simulink model "control_pos_6dof_sinMI"  (R2023b)
settings: Solver=ode45  StartTime=0.0  StopTime=tsim  FixedStep=tstep  MaxStep=tstep  RelTol=tstep/10
undefined symbols (not defined in the file): a0, a1, robot_params, t_qeq_init, t_tr_init, tau_L, tr_ref
(part 7 of 7)

== matlab function control_pos_6dof_sinMI/q to xyz (robot)/q to xyz ==
  data: robot_params input; p output size=[3,6]; q input size=[6,1]; dq input size=[6,1]; ddq input size=[6,1]; dp output size=[3,1]; ddp output size=[3,1]
function [p,dp,ddp] = fcn(robot_params,q,dq,ddq)

l1 = robot_params.l(1);
l2 = robot_params.l(2);
l3 = robot_params.l(3);
l4 = robot_params.l(4);
l5 = robot_params.l(5);
l6 = robot_params.l(6);

lc1 = robot_params.lc(1);
lc2 = robot_params.lc(2);
lc3 = robot_params.lc(3);
lc4 = robot_params.lc(4);
lc5 = robot_params.lc(5);
lc6 = robot_params.lc(6);

d1 = robot_params.d(1);
d2 = robot_params.d(2);
d3 = robot_params.d(3);
d4 = robot_params.d(4);
d5 = robot_params.d(5);
d6 = robot_params.d(6);

dc1 = robot_params.dc(1);
dc2 = robot_params.dc(2);
dc3 = robot_params.dc(3);
dc4 = robot_params.dc(4);
dc5 = robot_params.dc(5);
dc6 = robot_params.dc(6);

q1 = q(1);
q2 = q(2);
q3 = q(3);
q4 = q(4);
q5 = q(5);
q6 = q(6);


% Cinematica directa %%%%%%%%%%%%%%%%%%%%%%%%%%%%%%%%%%%%%%%%%%%%%%%%%%%%%%

DH = [0   pi/2  d1 q1;
      l2  0     0  q2;
      l3  0     0  q3;
      0   pi/2  d4 q4;
      0   -pi/2 d5 q5;
      0   0     d6 q6];

A01 = transformacion_homogenea(DH(1,:));
A12 = transformacion_homogenea(DH(2,:));
A23 = transformacion_homogenea(DH(3,:));
A34 = transformacion_homogenea(DH(4,:));
A45 = transformacion_homogenea(DH(5,:));
A56 = transformacion_homogenea(DH(6,:));

T0 = zeros(4,4,6);

T0(:,:,1) = A01;
T0(:,:,2) = A01*A12;
T0(:,:,3) = A01*A12*A23;
T0(:,:,4) = A01*A12*A23*A34;
T0(:,:,5) = A01*A12*A23*A34*A45;
T0(:,:,6) = A01*A12*A23*A34*A45*A56;

p = reshape(T0(1:3,4,:),[3,6]);


% Cinematica diferencial %%%%%%%%%%%%%%%%%%%%%%%%%%%%%%%%%%%%%%%%%%%%%%%%%%
JP = zeros(3,6);

JP(1,1) = -cos(q1)*(d1 + l3*sin(q2 + q3) + l2*sin(q2) - d5*cos(q2 + q3 + q4) - dc6*sin(q2 + q3 + q4)*sin(q5));
JP(1,2) = -cos(q1)*(d1 - dc1 + l3*sin(q2 + q3) + l2*sin(q2) - d5*cos(q2 + q3 + q4) - dc6*sin(q2 + q3 + q4)*sin(q5));
JP(1,3) = cos(q1)*(lc2*sin(q2) - l2*sin(q2) - l3*sin(q2 + q3) + d5*cos(q2 + q3 + q4) + dc6*sin(q2 + q3 + q4)*sin(q5));
JP(1,4) = - cos(q2 + q3 + q4)*(dc6*(cos(q1)*cos(q5) + cos(q2 + q3 + q4)*sin(q1)*sin(q5)) + d4*cos(q1) - sin(q1)*(l3*cos(q2 + q3) + l2*cos(q2)) + sin(q1)*(lc3*cos(q2 + q3) + l2*cos(q2)) - d5*sin(q2 + q3 + q4)*sin(q1)) - sin(q2 + q3 + q4)*sin(q1)*(lc3*sin(q2 + q3) - l3*sin(q2 + q3) + d5*cos(q2 + q3 + q4) + dc6*sin(q2 + q3 + q4)*sin(q5));
JP(1,5) = d5*sin(q1)*sin(q5) + d5*cos(q2 + q3 + q4)*cos(q1)*cos(q5) - d4*sin(q2 + q3 + q4)*cos(q1)*sin(q5) + dc4*sin(q2 + q3 + q4)*cos(q1)*sin(q5);
JP(1,6) = (d5 - dc5)*(sin(q1)*sin(q5) + cos(q2 + q3 + q4)*cos(q1)*cos(q5));

JP(2,1) = -sin(q1)*(d1 + l3*sin(q2 + q3) + l2*sin(q2) - d5*cos(q2 + q3 + q4) - dc6*sin(q2 + q3 + q4)*sin(q5));
JP(2,2) = -sin(q1)*(d1 - dc1 + l3*sin(q2 + q3) + l2*sin(q2) - d5*cos(q2 + q3 + q4) - dc6*sin(q2 + q3 + q4)*sin(q5));
JP(2,3) = sin(q1)*(lc2*sin(q2) - l2*sin(q2) - l3*sin(q2 + q3) + d5*cos(q2 + q3 + q4) + dc6*sin(q2 + q3 + q4)*sin(q5));
JP(2,4) = sin(q2 + q3 + q4)*cos(q1)*(lc3*sin(q2 + q3) - l3*sin(q2 + q3) + d5*cos(q2 + q3 + q4) + dc6*sin(q2 + q3 + q4)*sin(q5)) - cos(q2 + q3 + q4)*(dc6*(cos(q5)*sin(q1) - cos(q2 + q3 + q4)*cos(q1)*sin(q5)) + cos(q1)*(l3*cos(q2 + q3) + l2*cos(q2)) - cos(q1)*(lc3*cos(q2 + q3) + l2*cos(q2)) + d4*sin(q1) + d5*sin(q2 + q3 + q4)*cos(q1));
JP(2,5) = d5*cos(q2 + q3 + q4)*cos(q5)*sin(q1) - d5*cos(q1)*sin(q5) - d4*sin(q2 + q3 + q4)*sin(q1)*sin(q5) + dc4*sin(q2 + q3 + q4)*sin(q1)*sin(q5);
JP(2,6) = -(d5 - dc5)*(cos(q1)*sin(q5) - cos(q2 + q3 + q4)*cos(q5)*sin(q1));

JP(3,1) = l3*cos(q2 + q3) - (dc6*sin(q2 + q3 + q4 + q5))/2 + l2*cos(q2) + (dc6*sin(q2 + q3 + q4 - q5))/2 + d5*sin(q2 + q3 + q4);
JP(3,2) = l3*cos(q2 + q3) - (dc6*sin(q2 + q3 + q4 + q5))/2 + l2*cos(q2) + (dc6*sin(q2 + q3 + q4 - q5))/2 + d5*sin(q2 + q3 + q4);
JP(3,3) = l3*cos(q2 + q3) - (dc6*sin(q2 + q3 + q4 + q5))/2 + l2*cos(q2) - lc2*cos(q2) + (dc6*sin(q2 + q3 + q4 - q5))/2 + d5*sin(q2 + q3 + q4);
JP(3,4) = - (dc6*sin(q2 + q3 + q4 + q5))/2 - (dc6*sin(q2 + q3 + q4 - q5))/2 - d4*sin(q2 + q3 + q4);
JP(3,5) = d4*cos(q2 + q3 + q4)*sin(q5) + d5*sin(q2 + q3 + q4)*cos(q5) - dc4*cos(q2 + q3 + q4)*sin(q5);
JP(3,6) = sin(q2 + q3 + q4)*cos(q5)*(d5 - dc5);

dp = JP*dq;

dq1 = dq(1);
dq2 = dq(2);
dq3 = dq(3);

dJP = zeros(3,6);

dJP(1,1) = dq1*sin(q1)*(d1 + l3*sin(q2 + q3) + l2*sin(q2) - d5*cos(q2 + q3 + q4) - dc6*sin(q2 + q3 + q4)*sin(q5)) - dq3*cos(q1)*(l3*cos(q2 + q3) + d5*sin(q2 + q3 + q4) - dc6*cos(q2 + q3 + q4)*sin(q5)) - dq2*cos(q1)*(l3*cos(q2 + q3) + l2*cos(q2) + d5*sin(q2 + q3 + q4) - dc6*cos(q2 + q3 + q4)*sin(q5));
dJP(1,2) = dq1*sin(q1)*(d1 - dc1 + l3*sin(q2 + q3) + l2*sin(q2) - d5*cos(q2 + q3 + q4) - dc6*sin(q2 + q3 + q4)*sin(q5)) - dq3*cos(q1)*(l3*cos(q2 + q3) + d5*sin(q2 + q3 + q4) - dc6*cos(q2 + q3 + q4)*sin(q5)) - dq2*cos(q1)*(l3*cos(q2 + q3) + l2*cos(q2) + d5*sin(q2 + q3 + q4) - dc6*cos(q2 + q3 + q4)*sin(q5));
dJP(1,3) = - dq3*cos(q1)*(l3*cos(q2 + q3) + d5*sin(q2 + q3 + q4) - dc6*cos(q2 + q3 + q4)*sin(q5)) - dq2*cos(q1)*(l3*cos(q2 + q3) + l2*cos(q2) - lc2*cos(q2) + d5*sin(q2 + q3 + q4) - dc6*cos(q2 + q3 + q4)*sin(q5)) - dq1*sin(q1)*(lc2*sin(q2) - l2*sin(q2) - l3*sin(q2 + q3) + d5*cos(q2 + q3 + q4) + dc6*sin(q2 + q3 + q4)*sin(q5));
dJP(1,4) = dq1*l3*cos(q1)*cos(q4) - dq1*lc3*cos(q1)*cos(q4) - dc6*dq1*cos(q1)*sin(q5) + d4*dq1*cos(q2)*cos(q3)*cos(q4)*sin(q1) + d4*dq2*cos(q1)*cos(q2)*cos(q3)*sin(q4) + d4*dq2*cos(q1)*cos(q2)*cos(q4)*sin(q3) + d4*dq2*cos(q1)*cos(q3)*cos(q4)*sin(q2) + d4*dq3*cos(q1)*cos(q2)*cos(q3)*sin(q4) + d4*dq3*cos(q1)*cos(q2)*cos(q4)*sin(q3) + d4*dq3*cos(q1)*cos(q3)*cos(q4)*sin(q2) - d4*dq1*cos(q2)*sin(q1)*sin(q3)*sin(q4) - d4*dq1*cos(q3)*sin(q1)*sin(q2)*sin(q4) - d4*dq1*cos(q4)*sin(q1)*sin(q2)*sin(q3) - d4*dq2*cos(q1)*sin(q2)*sin(q3)*sin(q4) - d4*dq3*cos(q1)*sin(q2)*sin(q3)*sin(q4) + dc6*dq1*cos(q2)*cos(q3)*cos(q4)*cos(q5)*sin(q1) + dc6*dq2*cos(q1)*cos(q2)*cos(q3)*cos(q5)*sin(q4) + dc6*dq2*cos(q1)*cos(q2)*cos(q4)*cos(q5)*sin(q3) + dc6*dq2*cos(q1)*cos(q3)*cos(q4)*cos(q5)*sin(q2) + dc6*dq3*cos(q1)*cos(q2)*cos(q3)*cos(q5)*sin(q4) + dc6*dq3*cos(q1)*cos(q2)*cos(q4)*cos(q5)*sin(q3) + dc6*dq3*cos(q1)*cos(q3)*cos(q4)*cos(q5)*sin(q2) - dc6*dq1*cos(q2)*cos(q5)*sin(q1)*sin(q3)*sin(q4) - dc6*dq1*cos(q3)*cos(q5)*sin(q1)*sin(q2)*sin(q4) - dc6*dq1*cos(q4)*cos(q5)*sin(q1)*sin(q2)*sin(q3) - dc6*dq2*cos(q1)*cos(q5)*sin(q2)*sin(q3)*sin(q4) - dc6*dq3*cos(q1)*cos(q5)*sin(q2)*sin(q3)*sin(q4);
dJP(1,5) = dq1*(d5*cos(q1)*sin(q5) - d5*cos(q2 + q3 + q4)*cos(q5)*sin(q1) + d4*sin(q2 + q3 + q4)*sin(q1)*sin(q5) - dc4*sin(q2 + q3 + q4)*sin(q1)*sin(q5)) - dq2*cos(q1)*(d4*cos(q2 + q3 + q4)*sin(q5) + d5*sin(q2 + q3 + q4)*cos(q5) - dc4*cos(q2 + q3 + q4)*sin(q5)) - dq3*cos(q1)*(d4*cos(q2 + q3 + q4)*sin(q5) + d5*sin(q2 + q3 + q4)*cos(q5) - dc4*cos(q2 + q3 + q4)*sin(q5));
dJP(1,6) = dq1*(d5 - dc5)*(cos(q1)*sin(q5) - cos(q2 + q3 + q4)*cos(q5)*sin(q1)) - dq2*sin(q2 + q3 + q4)*cos(q1)*cos(q5)*(d5 - dc5) - dq3*sin(q2 + q3 + q4)*cos(q1)*cos(q5)*(d5 - dc5);

dJP(2,1) = - dq3*sin(q1)*(l3*cos(q2 + q3) + d5*sin(q2 + q3 + q4) - dc6*cos(q2 + q3 + q4)*sin(q5)) - dq1*cos(q1)*(d1 + l3*sin(q2 + q3) + l2*sin(q2) - d5*cos(q2 + q3 + q4) - dc6*sin(q2 + q3 + q4)*sin(q5)) - dq2*sin(q1)*(l3*cos(q2 + q3) + l2*cos(q2) + d5*sin(q2 + q3 + q4) - dc6*cos(q2 + q3 + q4)*sin(q5));
dJP(2,2) = - dq3*sin(q1)*(l3*cos(q2 + q3) + d5*sin(q2 + q3 + q4) - dc6*cos(q2 + q3 + q4)*sin(q5)) - dq2*sin(q1)*(l3*cos(q2 + q3) + l2*cos(q2) + d5*sin(q2 + q3 + q4) - dc6*cos(q2 + q3 + q4)*sin(q5)) - dq1*cos(q1)*(d1 - dc1 + l3*sin(q2 + q3) + l2*sin(q2) - d5*cos(q2 + q3 + q4) - dc6*sin(q2 + q3 + q4)*sin(q5));
dJP(2,3) = dq1*cos(q1)*(lc2*sin(q2) - l2*sin(q2) - l3*sin(q2 + q3) + d5*cos(q2 + q3 + q4) + dc6*sin(q2 + q3 + q4)*sin(q5)) - dq2*sin(q1)*(l3*cos(q2 + q3) + l2*cos(q2) - lc2*cos(q2) + d5*sin(q2 + q3 + q4) - dc6*cos(q2 + q3 + q4)*sin(q5)) - dq3*sin(q1)*(l3*cos(q2 + q3) + d5*sin(q2 + q3 + q4) - dc6*cos(q2 + q3 + q4)*sin(q5));
dJP(2,4) = dq1*l3*cos(q4)*sin(q1) - dq1*lc3*cos(q4)*sin(q1) - dc6*dq1*sin(q1)*sin(q5) - d4*dq1*cos(q1)*cos(q2)*cos(q3)*cos(q4) + d4*dq1*cos(q1)*cos(q2)*sin(q3)*sin(q4) + d4*dq1*cos(q1)*cos(q3)*sin(q2)*sin(q4) + d4*dq1*cos(q1)*cos(q4)*sin(q2)*sin(q3) + d4*dq2*cos(q2)*cos(q3)*sin(q1)*sin(q4) + d4*dq2*cos(q2)*cos(q4)*sin(q1)*sin(q3) + d4*dq2*cos(q3)*cos(q4)*sin(q1)*sin(q2) + d4*dq3*cos(q2)*cos(q3)*sin(q1)*sin(q4) + d4*dq3*cos(q2)*cos(q4)*sin(q1)*sin(q3) + d4*dq3*cos(q3)*cos(q4)*sin(q1)*sin(q2) - d4*dq2*sin(q1)*sin(q2)*sin(q3)*sin(q4) - d4*dq3*sin(q1)*sin(q2)*sin(q3)*sin(q4) - dc6*dq1*cos(q1)*cos(q2)*cos(q3)*cos(q4)*cos(q5) + dc6*dq1*cos(q1)*cos(q2)*cos(q5)*sin(q3)*sin(q4) + dc6*dq1*cos(q1)*cos(q3)*cos(q5)*sin(q2)*sin(q4) + dc6*dq1*cos(q1)*cos(q4)*cos(q5)*sin(q2)*sin(q3) + dc6*dq2*cos(q2)*cos(q3)*cos(q5)*sin(q1)*sin(q4) + dc6*dq2*cos(q2)*cos(q4)*cos(q5)*sin(q1)*sin(q3) + dc6*dq2*cos(q3)*cos(q4)*cos(q5)*sin(q1)*sin(q2) + dc6*dq3*cos(q2)*cos(q3)*cos(q5)*sin(q1)*sin(q4) + dc6*dq3*cos(q2)*cos(q4)*cos(q5)*sin(q1)*sin(q3) + dc6*dq3*cos(q3)*cos(q4)*cos(q5)*sin(q1)*sin(q2) - dc6*dq2*cos(q5)*sin(q1)*sin(q2)*sin(q3)*sin(q4) - dc6*dq3*cos(q5)*sin(q1)*sin(q2)*sin(q3)*sin(q4);
dJP(2,5) = dq1*(d5*sin(q1)*sin(q5) + d5*cos(q2 + q3 + q4)*cos(q1)*cos(q5) - d4*sin(q2 + q3 + q4)*cos(q1)*sin(q5) + dc4*sin(q2 + q3 + q4)*cos(q1)*sin(q5)) - dq2*sin(q1)*(d4*cos(q2 + q3 + q4)*sin(q5) + d5*sin(q2 + q3 + q4)*cos(q5) - dc4*cos(q2 + q3 + q4)*sin(q5)) - dq3*sin(q1)*(d4*cos(q2 + q3 + q4)*sin(q5) + d5*sin(q2 + q3 + q4)*cos(q5) - dc4*cos(q2 + q3 + q4)*sin(q5));
dJP(2,6) = dq1*(d5 - dc5)*(sin(q1)*sin(q5) + cos(q2 + q3 + q4)*cos(q1)*cos(q5)) - dq2*sin(q2 + q3 + q4)*cos(q5)*sin(q1)*(d5 - dc5) - dq3*sin(q2 + q3 + q4)*cos(q5)*sin(q1)*(d5 - dc5);

dJP(3,1) = - dq2*((dc6*cos(q2 + q3 + q4 + q5))/2 + l3*sin(q2 + q3) - (dc6*cos(q2 + q3 + q4 - q5))/2 + l2*sin(q2) - d5*cos(q2 + q3 + q4)) - dq3*((dc6*cos(q2 + q3 + q4 + q5))/2 + l3*sin(q2 + q3) - (dc6*cos(q2 + q3 + q4 - q5))/2 - d5*cos(q2 + q3 + q4));
dJP(3,2) = - dq2*((dc6*cos(q2 + q3 + q4 + q5))/2 + l3*sin(q2 + q3) - (dc6*cos(q2 + q3 + q4 - q5))/2 + l2*sin(q2) - d5*cos(q2 + q3 + q4)) - dq3*((dc6*cos(q2 + q3 + q4 + q5))/2 + l3*sin(q2 + q3) - (dc6*cos(q2 + q3 + q4 - q5))/2 - d5*cos(q2 + q3 + q4));
dJP(3,3) = - dq3*((dc6*cos(q2 + q3 + q4 + q5))/2 + l3*sin(q2 + q3) - (dc6*cos(q2 + q3 + q4 - q5))/2 - d5*cos(q2 + q3 + q4)) - dq2*((dc6*cos(q2 + q3 + q4 + q5))/2 + l3*sin(q2 + q3) - (dc6*cos(q2 + q3 + q4 - q5))/2 + l2*sin(q2) - lc2*sin(q2) - d5*cos(q2 + q3 + q4));
dJP(3,4) = -((dq2 + dq3)*(dc6*cos(q2 + q3 + q4 + q5) + dc6*cos(q2 + q3 + q4 - q5) + 2*d4*cos(q2 + q3 + q4)))/2;
dJP(3,5) = (dq2 + dq3)*(d5*cos(q2 + q3 + q4)*cos(q5) - d4*sin(q2 + q3 + q4)*sin(q5) + dc4*sin(q2 + q3 + q4)*sin(q5));
dJP(3,6) = cos(q2 + q3 + q4)*cos(q5)*(dq2 + dq3)*(d5 - dc5);

ddp = dJP*ddq;

end

function m = transformacion_homogenea(DH_i)
    a_i = DH_i(1);
    alpha_i = DH_i(2);
    d_i = DH_i(3);
    theta_i = DH_i(4);
    
    ma_i = [1 0 0 a_i;
            0 1 0 0;
            0 0 1 0;
            0 0 0 1];
    
    md_i = [1 0 0 0;
            0 1 0 0;
            0 0 1 d_i;
            0 0 0 1];
    
    mtheta_i = [cos(theta_i) -sin(theta_i) 0 0;
                sin(theta_i) cos(theta_i) 0 0;
                0 0 1 0;
                0 0 0 1];
    
    malpha_i = [1 0 0 0;
                0 cos(alpha_i) -sin(alpha_i) 0;
                0 sin(alpha_i) cos(alpha_i) 0;
                0 0 0 1];
    
    m = mtheta_i * md_i * ma_i * malpha_i;

end

== matlab function control_pos_6dof_sinMI/Inicializar posición de robot manipulador/dq_init/q3/Polinomio 7mo orden dq ==
  data: t input; q0 input; qpol output; vpol output; apol output; jpol output; q1 input; t0 input; t1 input
function [qpol,vpol,apol,jpol] = fcn(t,q0,q1,t0,t1)


% t,q0,q1,v0,v1,ac0,ac1,j0,j1,t0,t1)
%Trayectoria de referencia

% q0 = 0;
% q1 = 0;

v0 = 0;
v1 = 0;

ac0 = 0;
ac1 = 0;

j0 = 0;
j1 = 0;

% t0 = 0;
% t1 = pi/4;

% Coeficientes de un polinomio de 7mo grado

h = q1 - q0;
T = t1 - t0;

a = zeros(7+1,1);

a(1) = q0;
a(2) = v0;
a(3) = ac0/2;
a(4) = j0/6;
a(5) = (210*h-T*((30*ac0-15*ac1)*T+(4*j0+j1)*T^2+120*v0+90*v1))/(6*T^4);
a(6) = (-168*h-T*((20*ac0-14*ac1)*T+(2*j0+j1)*T^2+90*v0+78*v1))/(2*T^5);
a(7) = (420*h-T*((45*ac0-39*ac1)*T+(4*j0+3*j1)*T^2+216*v0+204*v1))/(6*T^6);
a(8) = (-120*h-T*((12*ac0-12*ac1)*T+(j0+j1)*T^2+60*v0+60*v1))/(6*T^7);

qa = flip(a')';
va = polyder(qa')';
aa = polyder(va')';
ja = polyder(aa')';


if t>=t0 && t<t1
    qpol = polyval(qa,t-t0);
    vpol = polyval(va,t-t0);
    apol = polyval(aa,t-t0);
    jpol = polyval(ja,t-t0);
elseif t>=t1
    qpol = polyval(qa,T);
    vpol = polyval(va,T);
    apol = polyval(aa,T);
    jpol = polyval(ja,T);
else
    qpol = q0;
    vpol = v0;
    apol = ac0;
    jpol = j0;
end

== matlab function control_pos_6dof_sinMI/xyz to q (referencia)/Cinemática inversa ==
  data: robot_params input; q output size=[6,1]; r input size=[3,1]; R input size=[3,3]
function q = fcn(robot_params,r,R)

%l1 = robot_params.l(1);
l2 = robot_params.l(2);
l3 = robot_params.l(3);
%l4 = robot_params.l(4);
%l5 = robot_params.l(5);
%l6 = robot_params.l(6);

d1 = robot_params.d(1);
%d2 = robot_params.d(2);
%d3 = robot_params.d(3);
d4 = robot_params.d(4);
d5 = robot_params.d(5);
d6 = robot_params.d(6);

Xr = r(1);
Yr = r(2);
Zr = r(3);

% Cinematica inversa %%%%%%%%%%%%%%%%%%%%%%%%%%%%%%%%%%%%%%%%%%%%%%%%%%%%%%

A = d6*R(2,3) - Yr;
B = Xr - d6*R(1,3);

q1 = - atan2(sqrt(B^2+A^2-d4^2),d4) + atan2(B,A); %signo

c1 = cos(q1);
s1 = sin(q1);

C = c1*R(1,1) + s1*R(2,1);
D = c1*R(2,2) - s1*R(1,2);
E = s1*R(1,1) - c1*R(2,1);

q5 = - atan2(sqrt(E^2+D^2),s1*R(1,3)-c1*R(2,3)); %signo

c5 = cos(q5);
s5 = sin(q5);

q6 = atan2(D/s5,E/s5);

c6 = cos(q6);
s6 = sin(q6);

F = c5*c6;  

q234 = atan2(R(3,1)*F-s6*C,F*C+s6*R(3,1));

c234 = cos(q234);
s234 = sin(q234);

KC = c1*Xr + s1*Yr - s234*d5 + c234*s5*d6;
KS = Zr - d1 + c234*d5 + s234*s5*d6;

c3 = (KS^2 + KC^2 - l2^2 - l3^2)/(2*l2*l3);
s3 = - sqrt(1-c3^2);

q3 = + atan2(s3,c3); %signo %no cambiar
q2 = atan2(KS,KC) - atan2(s3*l3,c3*l3+l2);
q4 = q234 - q2 - q3;


q = [q1;q2;q3;q4;q5;q6];
